simulink model "BLDC_regen_motor_control_VSI"  (R2023a)
settings: Solver=VariableStepAuto  StartTime=0.0  StopTime=10.0  RelTol=1e-3
undefined symbols (not defined in the file): Ion, Lithium
libraries: spsMeanLib x4, spsSeriesRLCBranchLib x2, spsVoltageMeasurementLib x2, spsBatteryLib x1, spsCurrentMeasurementLib x1, spsDCMachineLib x1, spsDCVoltageSourceLib x1, spsDiodeLib x1, spsMosfetLib x1, spsPWMGeneratorDCDCLib x1, spspowerguiLib x1
settings Model: Creator=sanja  LastModifiedBy=sanja

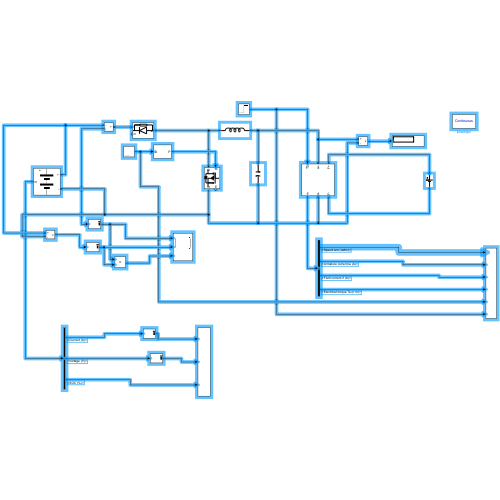
[thumbnail: Simulink's stored preview of the top-level diagram]
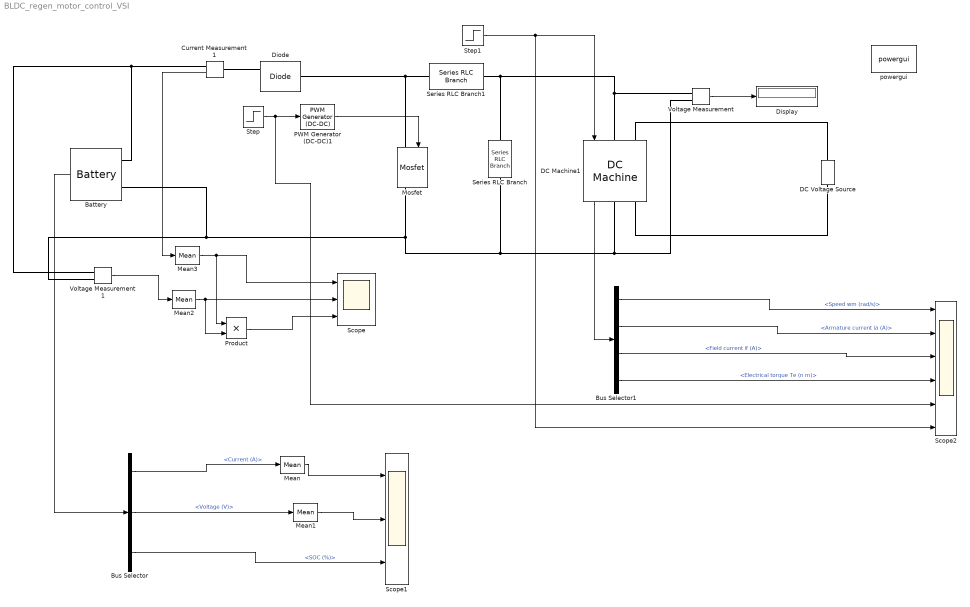
== system BLDC_regen_motor_control_VSI ==
  Battery : spsBatteryLib/Battery  BatType=Lithium-Ion  ShowTempParam=off  ThermalPreset=no  ShowAgeParam=off  NomV=240  NomQ=15.5  SOC=50  Batt_Tr=30  PresetModel=on  MaxQ=15.5  MinV=180  FullV=279.3569  Dis_rate=6.7391  R=0.15484  Normal_OP=14.0174  expZone="[259.2926     0.7615217]"  current=[6.5 13 32.5]  Units=Time  Tci=20  NomT=25  T2=0  MaxQ2=2.208  FullV2=3.45  Normal_OP2=2.8  expZone2="[3.22        0.23]"  Rca=0.6  ti=1000  Dp=0  Neq0=0  Tsim=1e6  Ta1=25  Qeol=5.4*0.9  Reol=0.013333*1.2  Char_age=[2.3478, 3]  Dis_age=[2.3478, 10]  N1=1500  N2=10500  N3=1000  N4=1400  Ta2=45  N5=950
      settings: LibrarySourceBlock=electricdrivelib/Extra Sources/Battery
  Bus Selector : BusSelector  OutputSignals=Current (A),Voltage (V),SOC (%)
  Bus Selector1 : BusSelector  OutputSignals=Speed wm (rad/s),Armature current ia (A),Field current if (A),Electrical torque Te (n m)
  Current Measurement1 : spsCurrentMeasurementLib/Current Measurement  PhasorSimulation=off  OutputType=Complex  PSBequivalent=0
  DC Machine1 : spsDCMachineLib/DC Machine  PresetModel=01: 5HP 240V 1750RPM Field:300V  MechanicalLoad=Torque TL  FieldType=Wound  ShowDetailedParameters=on  MeasurementBus=off  RLa=[2.581 0.028]  RLf=[281.2 156]  Laf=0.9483  MachineConstant=Torque constant (N.m/A)  Ke=1.8  Kt=1.8  J=0.02215  Bm=0.002953  Tf=0.5161  w0=1  Ifinit=1  TsPowergui=0  TsBlock=-1
  DC Voltage Source : spsDCVoltageSourceLib/DC Voltage Source  Amplitude=300  Measurements=None
  Diode : spsDiodeLib/Diode  Ron=0.001  Lon=0  Vf=0.8  IC=0  UseSnubber=off  Rs=500  Cs=250e-9  Measurements=on
  Display : Display
  Mean{,1..3} (4 alike) : spsMeanLib/Mean  Freq=60  Vinit=0  Ts=0
  Mosfet : spsMosfetLib/Mosfet  Ron=0.1  Lon=0  Rd=0.01  Vfd=0  IC=0  Rs=1e5  Cs=inf  Measurements=on
  PWM Generator (DC-DC)1 : spsPWMGeneratorDCDCLib/PWM Generator (DC-DC)  Fsw=5000  Ts=0
  Product : Product
  Scope : Scope  NumInputPorts=3
  Scope1 : Scope  NumInputPorts=3
  Scope2 : Scope  NumInputPorts=6
  Series RLC Branch : spsSeriesRLCBranchLib/Series RLC Branch  LConnTagsString=__new0  RConnTagsString=__new0  BranchType=C  Resistance=1  Inductance=1e-3  SetiL0=off  InitialCurrent=0  Capacitance=150e-6  Setx0=off  InitialVoltage=0  Measurements=None
  Series RLC Branch1 : spsSeriesRLCBranchLib/Series RLC Branch  LConnTagsString=__new0  RConnTagsString=__new0  BranchType=L  Resistance=1  Inductance=5e-3  SetiL0=off  InitialCurrent=0  Capacitance=1e-6  Setx0=off  InitialVoltage=0  Measurements=None
  Step : Step  Time=3  Before=0.6  After=0.8  SampleTime=0
  Step1 : Step  Time=7  Before=-20  After=-5  SampleTime=0
  Voltage Measurement : spsVoltageMeasurementLib/Voltage Measurement  PhasorSimulation=off  OutputType=Complex  PSBequivalent=0
  Voltage Measurement1 : spsVoltageMeasurementLib/Voltage Measurement  PhasorSimulation=off  OutputType=Complex  PSBequivalent=0
  powergui : spspowerguiLib/powergui  Priority=1  SimulationMode=Continuous  SampleTime=50e-6  frequency=60  Iterations=50  frequencyindice=0  Pbase=100e6  ErrMax=1e-4  UnitsV=kV  UnitsW=MW  buscounter=0  FunctionMessages=off  echomessages=off  EnableUseOfTLC=off  CurrentSourceSwitches=off  DisableSnubberDevices=off  DisableRonSwitches=off  DisableVfSwitches=off  DisplayEquations=off  AutomaticDiscreteSolvers=off  SolverType=Tustin/Backward Euler (TBE)  Interpol=off  ExternalGateDelay=off  methode=off  Ts=10  x0status=blocks  SPID=off  SwTol=0  HookPort=off  NonlinearTolerance=1e-4  nMaxIteration=100  ContinueOnMaxIteration=off  RestoreLinks=warning  ResistiveCurrentMeasurement=off  Frange=[0:2:500]  Ylog=off  Xlog=on  ShowGrid=off  save=off  variable=ZData  structure=0  ZoomFFT=off  StartTime=0.0  cycles=1  DisplayStyle=1  fundamental=60  FreqAxis=off  MaxFrequency=1000  frequencyindicesteady=1  RmsSteady=1  display=off
  wires:
  Mean2/1 -> Product/2, Scope/2
  Mean1/1 -> Scope1/2
  Bus Selector/3 -> Scope1/3  "<SOC (%)>"
  Step1/1 -> DC Machine1/1, Scope2/6
  Mean/1 -> Scope1/1
  Voltage Measurement/1 -> Display/1
  Bus Selector1/2 -> Scope2/2  "<Armature current ia (A)>"
  Product/1 -> Scope/3
  PWM Generator (DC-DC)1/1 -> Mosfet/1
  Bus Selector/2 -> Mean1/1  "<Voltage (V)>"
  Bus Selector/1 -> Mean/1  "<Current (A)>"
  Battery/1 -> Bus Selector/1
  DC Machine1/1 -> Bus Selector1/1
  Current Measurement1/1 -> Mean3/1
  Bus Selector1/4 -> Scope2/4  "<Electrical torque Te (n m)>"
  Voltage Measurement1/1 -> Mean2/1
  Step/1 -> PWM Generator (DC-DC)1/1, Scope2/5
  Mean3/1 -> Product/1, Scope/1
  Bus Selector1/3 -> Scope2/3  "<Field current if (A)>"
  Bus Selector1/1 -> Scope2/1  "<Speed wm (rad/s)>"
  connections:
  Voltage Measurement1/LConn1 -- Current Measurement1/RConn1 -- Battery/LConn1
  Series RLC Branch/LConn1 -- Series RLC Branch1/RConn1 -- DC Machine1/LConn1 -- Voltage Measurement/LConn1
  Series RLC Branch/RConn1 -- DC Machine1/RConn1 -- Voltage Measurement/LConn2 -- Battery/LConn2 -- Voltage Measurement1/LConn2 -- Mosfet/RConn1
  Mosfet/LConn1 -- Series RLC Branch1/LConn1 -- Diode/LConn1
  Current Measurement1/LConn1 -- Diode/RConn1
  DC Machine1/LConn2 -- DC Voltage Source/RConn1
  DC Voltage Source/LConn1 -- DC Machine1/RConn2
